simulink model "sine_dyn"  (R2022a)
settings: Solver=VariableStepAuto  StartTime=0.0  StopTime=12  MaxStep=0.05  RelTol=1e-3
libraries: simulink x2
settings Model: Creator=patri  LastModifiedBy=Mattia
settings SolverCC: ZeroCrossAlgorithm=Adaptive
settings DebuggingCC: IgnoredZcDiagnostic=none

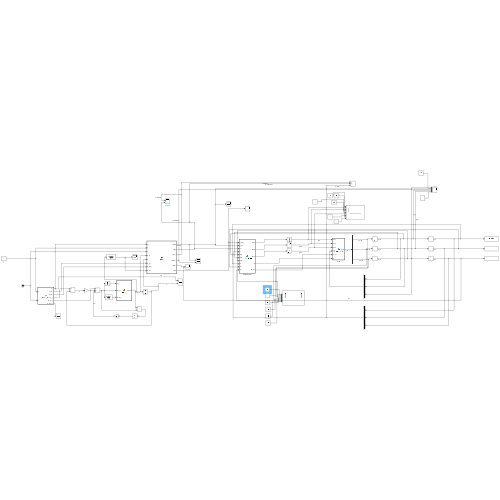
[thumbnail: Simulink's stored preview of the top-level diagram]
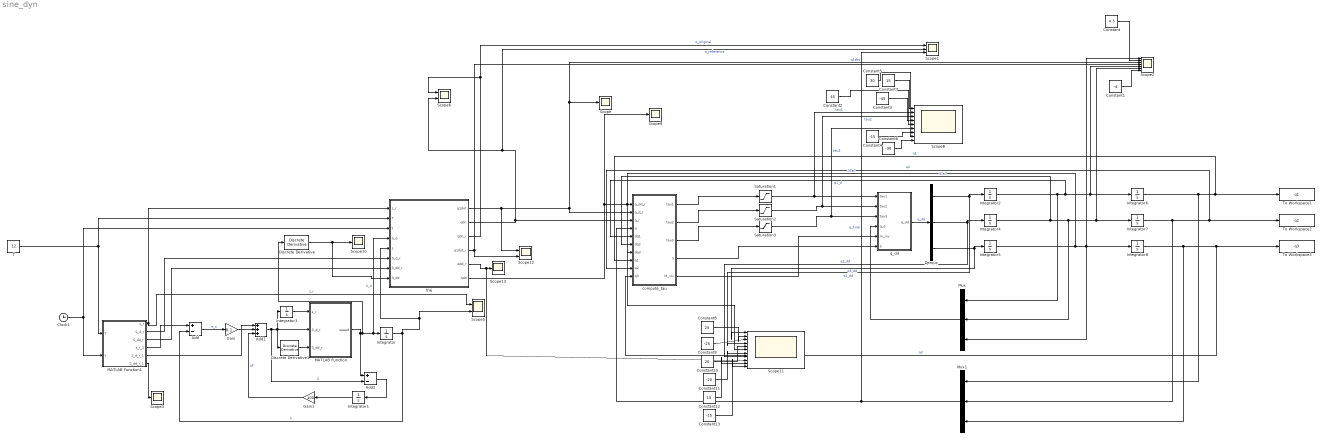
== system sine_dyn ==
  Add : Sum  Inputs=+-
  Add1 : Sum  Inputs=+++
  Add2 : Sum  Inputs=+-
  Clock1 : Clock
  Constant : Constant  Value=4.3
  Constant1 : Constant  Value=-4
  Constant10 : Constant  Value=20
  Constant11 : Constant  Value=-20
  Constant12 : Constant  Value=15
  Constant13 : Constant  Value=-15
  Constant2 : Constant  Value=45
  Constant3 : Constant  Value=-45
  Constant4 : Constant  Value=-15
  Constant5 : Constant  Value=30
  Constant6 : Constant  Value=-30
  Constant7 : Constant  Value=15
  Constant8 : Constant  Value=25
  Constant9 : Constant  Value=-25
  Demux : Demux  Outputs=3
  Discrete Derivative : simulink/Discrete/Discrete Derivative  gainval=1.0  ICPrevScaledInput=0.0  OutMin=[]  OutMax=[]  OutDataType=fixdt(1, 16)  OutScaling=2^-10  DoSatur=off
  Discrete Derivative1 : simulink/Discrete/Discrete Derivative  gainval=1.0  ICPrevScaledInput=0.0  OutMin=[]  OutMax=[]  OutDataType=fixdt(1, 16)  OutScaling=2^-10  DoSatur=off
  Gain : Gain  Gain=0.1
  Gain1 : Gain  Gain=100
  Integrator{,1..5} (6 alike) : Integrator
  Integrator6 : Integrator  InitialCondition=2.6180
  Integrator7 : Integrator  InitialCondition=-2.0944
  Integrator8 : Integrator  InitialCondition=-0.5236
  MATLAB Function : MATLAB Function  TreatAsAtomicUnit=on
  MATLAB Function1 : MATLAB Function  TreatAsAtomicUnit=on
  Mux : Mux  Inputs=3
  Mux1 : Mux  Inputs=3
  Saturation1 : Saturate  UpperLimit=45  LowerLimit=-45  LinearizeAsGain=off  ZeroCross=off
  Saturation2 : Saturate  UpperLimit=30  LowerLimit=-30  LinearizeAsGain=off  ZeroCross=off
  Saturation3 : Saturate  UpperLimit=15  LowerLimit=-15  LinearizeAsGain=off  ZeroCross=off
  Scope{,3,9..10,13} (5 alike) : Scope
  Scope1 : Scope  NumInputPorts=3
  Scope11 : Scope  NumInputPorts=11
  Scope12 : Scope  NumInputPorts=2
  Scope2 : Scope  NumInputPorts=7
  Scope5 : Scope  NumInputPorts=2
  Scope6 : Scope  NumInputPorts=2
  Scope8 : Scope  NumInputPorts=9
  T : Constant  Value=12
  To Workspace1 : ToWorkspace  VariableName=q1  SampleTime=-1
  To Workspace2 : ToWorkspace  VariableName=q2  SampleTime=-1
  To Workspace3 : ToWorkspace  VariableName=q3  SampleTime=-1
  compute_tau : MATLAB Function  TreatAsAtomicUnit=on
  q_dd : MATLAB Function  TreatAsAtomicUnit=on
  traj : MATLAB Function  TreatAsAtomicUnit=on
  wires:
  Demux/3 -> Integrator5/1, Scope11/1  "q3_dd"
  traj/2(q0n) -> compute_tau/3(q_r), Scope1/2, Scope6/2  "q_reference"
  Clock1/1 -> MATLAB Function1/2(t), traj/3(t)
  q_dd/1(q_dd) -> Demux/1  "q_dd"
  traj/3(q0n_r) -> Scope1/1, Scope6/1  "q_original"
  Add2/1 -> Integrator1/1
  Integrator4/1 -> compute_tau/6(dq2), Mux/2, Integrator7/1, Scope2/6  "q2_d"
  Integrator/1 -> traj/5(s), Scope5/2, Add/2  "s"
  compute_tau/4(S) -> q_dd/6(S)
  Integrator5/1 -> compute_tau/7(dq3), Scope2/1, Mux/3, Integrator8/1  "q3_d"
  Mux/1 -> q_dd/4(q_d)
  Demux/1 -> Integrator2/1, Scope11/4  "q1_dd"
  Mux1/1 -> Scope1/3, compute_tau/4(q)  "q_final"
  Integrator2/1 -> Mux/1, compute_tau/5(dq1), Scope2/5, Integrator6/1  "q1_d"
  Integrator6/1 -> Mux1/1, compute_tau/8(q1), To Workspace1/1  "q1"
  traj/6(qdd) -> Scope9/1, compute_tau/1(q_dd_r), Scope11/6
  MATLAB Function1/1(s_r) -> traj/1(s_r), Scope5/1  "s_r"
  Integrator8/1 -> Mux1/3, To Workspace3/1, compute_tau/10(q3)  "q3"
  traj/1(q1dot) -> Scope12/1, Scope2/3, Scope/1, compute_tau/2(q_d_r)  "q1dot"
  Gain/1 -> Add1/2
  compute_tau/5(M_inv) -> q_dd/5(m_inv)
  Add1/1 -> Add2/2, MATLAB Function/2(S_d_r), Discrete Derivative1/1, Integrator3/1  "U"
  T/1 -> MATLAB Function1/1(T), traj/2(T)
  MATLAB Function/1(speed) -> Add2/1, Discrete Derivative/1, traj/4(S_d), Integrator/1  "S_d"
  Add/1 -> Gain/1  "e_s"
  Gain1/1 -> Add1/3  "Uf"
  traj/4(q1dot_r) -> Scope2/4, Scope12/2
  Demux/2 -> Integrator4/1, Scope11/8  "q2_dd"
  Integrator1/1 -> Gain1/1
  Integrator7/1 -> Mux1/2, compute_tau/9(q2), To Workspace2/1  "q2"
  compute_tau/1(tau1) -> Saturation1/1
  Saturation1/1 -> Scope8/2, q_dd/1(tau1)  "tau1"
  compute_tau/2(tau2) -> Saturation2/1
  Saturation2/1 -> Scope8/3, q_dd/2(tau2)  "tau2"
  compute_tau/3(tau3) -> Saturation3/1
  Saturation3/1 -> Scope8/6, q_dd/3(tau3)  "tau3"
  Constant1/1 -> Scope2/7
  Constant/1 -> Scope2/2
  MATLAB Function1/2(S_d_r) -> traj/6(S_d_r)
  MATLAB Function1/3(S_dd_r) -> traj/7(S_dd_r)
  Constant4/1 -> Scope8/7
  Constant3/1 -> Scope8/4
  Constant7/1 -> Scope8/1
  Constant2/1 -> Scope8/5
  Discrete Derivative/1 -> Scope10/1, traj/8(S_dd)
  traj/5(qdd_r) -> Scope11/9, Scope13/1
  MATLAB Function1/4(s_r_1) -> Add/1
  MATLAB Function1/5(S_d_r_1) -> Add1/1
  MATLAB Function1/6(S_dd_r_1) -> Scope3/1
  Integrator3/1 -> MATLAB Function/1(s_r)
  Discrete Derivative1/1 -> MATLAB Function/3(S_dd_r)
  Constant5/1 -> Scope8/8
  Constant6/1 -> Scope8/9
  Constant8/1 -> Scope11/2
  Constant9/1 -> Scope11/3
  Constant10/1 -> Scope11/5
  Constant11/1 -> Scope11/7
  Constant12/1 -> Scope11/10
  Constant13/1 -> Scope11/11

== matlab function sine_dyn/q_dd ==
  data: tau1 input; tau2 input; tau3 input; q_dd output; q_d input; m_inv input; S input
function q_dd = compute_q_dd(tau1,tau2,tau3,q_d,m_inv,S)

tau = [tau1;
       tau2;
       tau3];
q_dd = m_inv*(tau - (S*q_d));

== matlab function sine_dyn/compute_tau ==
  data: q_dd_r input; tau1 output; tau2 output; tau3 output; q_d_r input; q_r input; q input; dq1 input; S output; M_inv output; dq2 input; dq3 input; q1 input; q2 input; q3 input
function [tau1,tau2,tau3,S,M_inv] = compute_tau(q_dd_r, q_d_r, q_r, q,dq1,dq2,dq3,q1,q2,q3)

% M(q)q_dd_r + S(q,q_d)q_d_r + Kp(q_r - q) + Kd (q_d_r - q_d)

% 
Kp = diag([0.1,0.1,0.1]);

Kd= diag([10,10,10]);

% 
%NEW GAIN TO STABILIZE ACCELERATION
% Kp = diag([30,30,30]);
% 
% Kd = diag([100,100,100]);

%%q

% q1=q_r(1);
% q2=q_r(2);
% q3=q_r(3);
% %%dq
% dq1=q_d_r(1);
% dq2=q_d_r(2);
% dq3=q_d_r(3);

q_d = [dq1;dq2;dq3];

%%position error
e = q_r - q;
%%velocity error
e_d = q_d_r - q_d;

L=1;

l1 = L;
l2 = L;
l3 = L;
dc1 = 1/2 * L;
dc2 = 1/2 * L;
dc3 = 1/2 * L;
m1 = 5;
m2 = 5;
m3 = 5;
I1 = 1/12 * m1 * L^2;
I2 = 1/12 * m2 * L^2;
I3 = 1/12 * m3 * L^2;

M=zeros(3,3);

M(1,1)=I1 + I2 + I3 + L^2*m2 + 2*L^2*m3 + 2*cos(q2)*(m3*L^2 + dc2*m2*L) + dc1^2*m1 + dc2^2*m2 + dc3^2*m3 + 2*L*dc3*m3*cos(q2 + q3) + 2*L*dc3*m3*cos(q3);
M(1,2)=I2 + I3 + L^2*m3 + cos(q2)*(m3*L^2 + dc2*m2*L) + dc2^2*m2 + dc3^2*m3 + L*dc3*m3*cos(q2 + q3) + 2*L*dc3*m3*cos(q3);
M(1,3)=I3 + dc3^2*m3 + L*dc3*m3*cos(q2 + q3) + L*dc3*m3*cos(q3);
M(2,2)=m3*L^2 + 2*m3*cos(q3)*L*dc3 + m2*dc2^2 + m3*dc3^2 + I2 + I3;
M(2,3)=m3*dc3^2 + L*m3*cos(q3)*dc3 + I3;
M(3,3)=m3*dc3^2 + I3;
M(2,1)=M(1,2);
M(3,1)=M(1,3);
M(3,2)=M(2,3);

M_inv = pinv(M);

S=zeros(3,3);

S(1,1) = -dq2*(dc3*l1*m3*sin(q2 + q3) + dc2*l1*m2*sin(q2) + l1*l2*m3*sin(q2)) - dq3*(dc3*l1*m3*sin(q2 + q3) + dc3*l2*m3*sin(q3));

S(1,2)= -dq1*(dc3*l1*m3*sin(q2 + q3) + dc2*l1*m2*sin(q2) + l1*l2*m3*sin(q2)) - dq2*(dc3*l1*m3*sin(q2 + q3) + dc2*l1*m2*sin(q2) + l1*l2*m3*sin(q2)) - dq3*(dc3*l1*m3*sin(q2 + q3) + dc3*l2*m3*sin(q3));

S(1,3)= -dq1*(dc3*l1*m3*sin(q2 + q3) + dc3*l2*m3*sin(q3)) - dq2*(dc3*l1*m3*sin(q2 + q3) + dc3*l2*m3*sin(q3)) - dq3*(dc3*l1*m3*sin(q2 + q3) + dc3*l2*m3*sin(q3)) ;

S(2,1)= dq1*(dc3*l1*m3*sin(q2 + q3) + dc2*l1*m2*sin(q2) + l1*l2*m3*sin(q2)) - dc3*dq3*l2*m3*sin(q3);

S(2,2)=-dc3*dq3*l2*m3*sin(q3);
 
S(2,3)= - dc3*dq1*l2*m3*sin(q3) - dc3*dq2*l2*m3*sin(q3) - dc3*dq3*l2*m3*sin(q3);

S(3,1)= dq1*(dc3*l1*m3*sin(q2 + q3) + dc3*l2*m3*sin(q3)) + dc3*dq2*l2*m3*sin(q3);

S(3,2)= dc3*dq1*l2*m3*sin(q3) + dc3*dq2*l2*m3*sin(q3);

S(3,3)= 0;


%torque = M*q_dd_r + S*q_d_r + Kp*e + Kd*e_d; %%viscous friction Fv*q_d_r
torque =M*q_dd_r + S*q_d_r + M*(Kp*e + Kd*e_d);

tau1 = torque(1);
tau2 = torque(2);
tau3 = torque(3);



%torque = M(q)*q_dd_r + S(q,q_d)*q_d_r + Kp*(q_r - q) + Kd*(q_d_r - q_d);

== matlab function sine_dyn/MATLAB Function1 ==
  data: T input; t input; s_r output; S_d_r output; S_dd_r output; s_r_1 output; S_d_r_1 output; S_dd_r_1 output
function [s_r, S_d_r, S_dd_r,s_r_1, S_d_r_1, S_dd_r_1] = timing_law(T, t)

tau_t=t/T;
%s_r = -2*tau_t^3 + 3*tau_t^2;
s_r = 10*tau_t^3 - 15*tau_t^4 + 6*tau_t^5;
S_d_r = (30*t^2)/T^3 - (60*t^3)/T^4 + (30*t^4)/T^5;
S_dd_r=(60*t)/T^3 - (180*t^2)/T^4 + (120*t^3)/T^5;
t_1 = t +0.0001;
tau_t_1 = t_1/T;
s_r_1 = 10*tau_t_1^3 - 15*tau_t_1^4 + 6*tau_t_1^5;
S_d_r_1 = (30*t_1^2)/T^3 - (60*t_1^3)/T^4 + (30*t_1^4)/T^5;
S_dd_r_1=(60*t_1)/T^3 - (180*t_1^2)/T^4 + (120*t_1^3)/T^5;

== matlab function sine_dyn/traj ==
  data: s_r input; T input; t input; S_d input; s input; q1dot output; q0n output; q0n_r output; q1dot_r output; S_d_r input; S_dd_r input; qdd_r output; qdd output; S_dd input
function [q1dot,q0n,q0n_r,q1dot_r, qdd_r, qdd] = trajectory(s_r, T, t, S_d, s, S_d_r, S_dd_r, S_dd)


%Links length
l1 = 1; l2 =1; l3 = 1;

%Trajectory

p_s = [s + 1;
    1 + sin(4*pi*s);
    s];

p_s_r =  [s_r + 1;
    1 + sin(4*pi*s_r);
    s_r];

p1_s=[1;
        4*pi*cos(4*pi*s);
        1];
p1_s_r=[1;
        4*pi*cos(4*pi*s_r);
        1];

%Velocity of the trajectory
pdot_s= p1_s* S_d ;
pdot_s_r = p1_s_r * S_d_r;
                                                                 

%End effector position
px = p_s(1); py = p_s(2); %position of the end effector w.r.t. the global frame

phi = p_s(3); %orientation of the end effector w.r.t. global frame

%%% REFERENCE

px_r=p_s_r(1); py_r = p_s_r(2);
phi_r = p_s_r(3);

%%Inverse kinematics of planar 3R
%fprintf("we first solve the joint variables q1, q2 in order to place\nthe position of the base of the third link in the necessary position\n");
 
p2 = [px; py] - [l3*cos(phi); l3*sin(phi)];
p2x = p2(1);
p2y = p2(2);

%%% REFERENCE

p2_r = [px_r; py_r] - [l3*cos(phi_r); l3*sin(phi_r)];
p2x_r = p2_r(1);
p2y_r = p2_r(2);

% second joint computations
c2=(p2x^2+p2y^2-l1^2-l2^2)/(2*l1*l2); s2pos=sqrt(1-c2^2);

%%% REFERENCE

c2_r=(p2x_r^2+p2y_r^2-l1^2-l2^2)/(2*l1*l2); s2pos_r=sqrt(1-c2_r^2);

%other solution: -sqrt(1-c2^2)
s2neg=-sqrt(1-c2^2);

q02p=atan2(s2pos,c2);
q02n=atan2(s2neg,c2);

%%% REFERENCE

s2neg_r=-sqrt(1-c2_r^2);

q02p_r=atan2(s2pos_r,c2_r);
q02n_r=atan2(s2neg_r,c2_r);
 
% first joint computations
detM=l1^2+l2^2+2*l1*l2*c2;

%%% REFERENCE

detM_r=l1^2+l2^2+2*l1*l2*c2_r;

% positive solution of q1
s1pos=(p2y*(l1+l2*c2)-p2x*l2*s2pos)/detM; c1pos=(p2x*(l1+l2*c2)+p2y*l2*s2pos)/detM;

%%% REFERENCE

s1pos_r=(p2y_r*(l1+l2*c2_r)-p2x_r*l2*s2pos_r)/detM_r; c1pos_r=(p2x_r*(l1+l2*c2_r)+p2y_r*l2*s2pos_r)/detM_r;

% negative solution of q1
s1neg=(p2y*(l1+l2*c2)-p2x*l2*s2neg)/detM;
c1neg=(p2x*(l1+l2*c2)+p2y*l2*s2neg)/detM;

q01p=atan2(s1pos,c1pos);
q01n=atan2(s1neg,c1neg); 

q03p = phi-(q01p+q02p);
q03n = phi-(q01n+q02n);

%%% REFERENCE

s1neg_r=(p2y_r*(l1+l2*c2_r)-p2x_r*l2*s2neg_r)/detM_r;
c1neg_r=(p2x_r*(l1+l2*c2_r)+p2y_r*l2*s2neg_r)/detM_r;

q01p_r=atan2(s1pos_r,c1pos_r);
q01n_r=atan2(s1neg_r,c1neg_r); 

q03p_r = phi_r-(q01p_r+q02p_r);
q03n_r = phi_r-(q01n_r+q02n_r);

% output positive
q0p=[q01p; q02p; q03p];

%%% REFERENCE

q0p_r=[q01p_r; q02p_r; q03p_r];
% output negative
q0n=[q01n; q02n; q03n];

%%% REFERENCE

q0n_r=[q01n_r; q02n_r; q03n_r];

%In a cubic polynomial the maximum of the speed of the timing law is
%obtained in t = T/2 
q1 = q0n(1);
q2 = q0n(2);
q3 = q0n(3);
P = [l1*cos(q1) + l2*cos(q1+q2) + l3*cos(q1+q2+q3);
    l1*sin(q1) + l2*sin(q1+q2) + l3*sin(q1+q2+q3)
    q1 + q2 + q3];

J = [- sin(q1 + q2 + q3) - sin(q1 + q2) - sin(q1), - sin(q1 + q2 + q3) - sin(q1 + q2), -sin(q1 + q2 + q3);
  cos(q1 + q2 + q3) + cos(q1 + q2) + cos(q1),   cos(q1 + q2 + q3) + cos(q1 + q2),  cos(q1 + q2 + q3);
                                          1,                                  1,                  1];

%%% REFERENCE

q1_r = q0n_r(1);
q2_r = q0n_r(2);
q3_r = q0n_r(3);
P_r = [l1*cos(q1_r) + l2*cos(q1_r+q2_r) + l3*cos(q1_r+q2_r+q3_r);
    l1*sin(q1_r) + l2*sin(q1_r+q2_r) + l3*sin(q1_r+q2_r+q3_r)
    q1 + q2 + q3];

J_r = [- sin(q1_r + q2_r + q3_r) - sin(q1_r + q2_r) - sin(q1_r), - sin(q1_r + q2_r + q3_r) - sin(q1_r + q2_r), -sin(q1_r + q2_r + q3_r);
  cos(q1_r + q2_r + q3_r) + cos(q1_r + q2_r) + cos(q1_r),   cos(q1_r + q2_r + q3_r) + cos(q1_r + q2_r),  cos(q1_r + q2_r + q3_r);
                                          1,                                  1,                  1];


qdot = pinv(J) * pdot_s;

%%% REFERENCE

qdot_r = pinv(J_r) * pdot_s_r;

q1dot = qdot;

q1dot_r = qdot_r;

dq1_r=qdot_r(1);
dq2_r=qdot_r(2);
dq3_r=qdot_r(3);
J_dot_r = [- cos(q1_r + q2_r + q3_r)*(dq1_r + dq2_r + dq3_r) - cos(q1_r + q2_r)*(dq1_r + dq2_r) - dq1_r*cos(q1_r), - cos(q1_r + q2_r + q3_r)*(dq1_r + dq2_r + dq3_r) - cos(q1_r + q2_r)*(dq1_r + dq2_r), -cos(q1_r + q2_r + q3_r)*(dq1_r + dq2_r + dq3_r);
           - sin(q1_r + q2_r + q3_r)*(dq1_r + dq2_r + dq3_r) - sin(q1_r + q2_r)*(dq1_r + dq2_r) - dq1_r*sin(q1_r), - sin(q1_r + q2_r + q3_r)*(dq1_r + dq2_r + dq3_r) - sin(q1_r + q2_r)*(dq1_r + dq2_r), -sin(q1_r + q2_r + q3_r)*(dq1_r + dq2_r + dq3_r) ;   
            0,0,0];
p2_s_r =[   0
-16*pi^2*sin(4*pi*s_r)
                     0];
p2_s =[   0
-16*pi^2*sin(4*pi*s)
                     0];
dq1=qdot(1);
dq2=qdot(2);
dq3=qdot(3);
J_dot = [- cos(q1 + q2 + q3)*(dq1 + dq2 + dq3) - cos(q1 + q2)*(dq1 + dq2) - dq1*cos(q1), - cos(q1 + q2 + q3)*(dq1 + dq2 + dq3) - cos(q1 + q2)*(dq1 + dq2), -cos(q1 + q2 + q3)*(dq1 + dq2 + dq3);
    - sin(q1 + q2 + q3)*(dq1 + dq2 + dq3) - sin(q1 + q2)*(dq1 + dq2) - dq1*sin(q1), - sin(q1 + q2 + q3)*(dq1 + dq2 + dq3) - sin(q1 + q2)*(dq1 + dq2), -sin(q1 + q2 + q3)*(dq1 + dq2 + dq3);
    0,0,0];

pdd_r = p1_s_r * S_dd_r + p2_s_r * S_d_r^2;

qdd_r = inv(J_r)*(pdd_r - J_dot_r*qdot_r);
pdd = p1_s * S_dd + p2_s * S_d^2;


qdd = inv(J)*(pdd - J_dot*qdot);

== matlab function sine_dyn/MATLAB Function ==
  data: s_r input; speed output; S_d_r input; S_dd_r input
function speed = trajectory(s_r, S_d_r,S_dd_r)

%Links length
l1 = 1; l2 =1; l3 = 1;

%Trajectory


%%% REFERENCE


p_s_r =  [s_r + 1;
    1 + sin(4*pi*s_r);
    s_r];

R1_s_r=[1;
        4*pi*cos(4*pi*s_r);
        1];

%Velocity of the trajectory


%%pdot = R'*s'(t)




%%% REFERENCE

%%%POLYNOMIAL OF DEGREE 5 ---  0.4808 saturation --- 3.9 seconds
% pdot_s_r=[ -(30*t^2*pi*sin((2*t^3*pi*(10*T^2 - 15*T*t + 6*t^2))/T^5)*(T - t)^2)/T^5;
%           (30*t^2*pi*cos((2*t^3*pi*(10*T^2 - 15*T*t + 6*t^2))/T^5)*(T - t)^2)/T^5;
%                                                                                 0];
pdot_s_r= R1_s_r* S_d_r ; %sdr is u
      

%%%%%%%%%%%%%%%%%%%
% pdot_s_r = [-pi*sin(2*pi*((10*t^3)/T^3 - (15*t^4)/T^4 + (6*t^5)/T^5))*((30*t^2)/T^3 - (60*t^3)/T^4 + (30*t^4)/T^5);
%  pi*cos(2*pi*((10*t^3)/T^3 - (15*t^4)/T^4 + (6*t^5)/T^5))*((30*t^2)/T^3 - (60*t^3)/T^4 + (30*t^4)/T^5);
%                                                                                                      0];

%End effector position

%%% REFERENCE

px_r=p_s_r(1); py_r = p_s_r(2);
phi_r = p_s_r(3);

%%Inverse kinematics of planar 3R, compute q

%%% REFERENCE

p2_r = [px_r; py_r] - [l3*cos(phi_r); l3*sin(phi_r)];
p2x_r = p2_r(1);
p2y_r = p2_r(2);

% second joint computations


%%% REFERENCE

c2_r=(p2x_r^2+p2y_r^2-l1^2-l2^2)/(2*l1*l2); s2pos_r=sqrt(1-c2_r^2);

%other solution: -sqrt(1-c2^2)

%%% REFERENCE

s2neg_r=-sqrt(1-c2_r^2);

q02p_r=atan2(s2pos_r,c2_r);
q02n_r=atan2(s2neg_r,c2_r);
 
% first joint computations


%%% REFERENCE

detM_r=l1^2+l2^2+2*l1*l2*c2_r;

% positive solution of q1


%%% REFERENCE

s1pos_r=(p2y_r*(l1+l2*c2_r)-p2x_r*l2*s2pos_r)/detM_r; c1pos_r=(p2x_r*(l1+l2*c2_r)+p2y_r*l2*s2pos_r)/detM_r;

% negative solution of q1


%%% REFERENCE

s1neg_r=(p2y_r*(l1+l2*c2_r)-p2x_r*l2*s2neg_r)/detM_r;
c1neg_r=(p2x_r*(l1+l2*c2_r)+p2y_r*l2*s2neg_r)/detM_r;

q01p_r=atan2(s1pos_r,c1pos_r);
q01n_r=atan2(s1neg_r,c1neg_r); 

q03p_r = phi_r-(q01p_r+q02p_r);
q03n_r = phi_r-(q01n_r+q02n_r);



%%% REFERENCE


% output negative


%%% REFERENCE

q0n_r=[q01n_r; q02n_r; q03n_r];
q1_r = q0n_r(1);
q2_r = q0n_r(2);
q3_r = q0n_r(3);

%NOW WE COMPUTE qdot, qdotdot

%%% REFERENCE


P_r = [l1*cos(q1_r) + l2*cos(q1_r+q2_r) + l3*cos(q1_r+q2_r+q3_r);
    l1*sin(q1_r) + l2*sin(q1_r+q2_r) + l3*sin(q1_r+q2_r+q3_r)
    q1_r + q2_r + q3_r];

J_r = [- sin(q1_r + q2_r + q3_r) - sin(q1_r + q2_r) - sin(q1_r), - sin(q1_r + q2_r + q3_r) - sin(q1_r + q2_r), -sin(q1_r + q2_r + q3_r);
  cos(q1_r + q2_r + q3_r) + cos(q1_r + q2_r) + cos(q1_r),   cos(q1_r + q2_r + q3_r) + cos(q1_r + q2_r),  cos(q1_r + q2_r + q3_r);
                                          1,                                  1,                  1];


qdot_r = pinv(J_r) * pdot_s_r;

dq1_r=qdot_r(1);
dq2_r=qdot_r(2);
dq3_r=qdot_r(3);
J_dot_r = [- cos(q1_r + q2_r + q3_r)*(dq1_r + dq2_r + dq3_r) - cos(q1_r + q2_r)*(dq1_r + dq2_r) - dq1_r*cos(q1_r), - cos(q1_r + q2_r + q3_r)*(dq1_r + dq2_r + dq3_r) - cos(q1_r + q2_r)*(dq1_r + dq2_r), -cos(q1_r + q2_r + q3_r)*(dq1_r + dq2_r + dq3_r);
           - sin(q1_r + q2_r + q3_r)*(dq1_r + dq2_r + dq3_r) - sin(q1_r + q2_r)*(dq1_r + dq2_r) - dq1_r*sin(q1_r), - sin(q1_r + q2_r + q3_r)*(dq1_r + dq2_r + dq3_r) - sin(q1_r + q2_r)*(dq1_r + dq2_r), -sin(q1_r + q2_r + q3_r)*(dq1_r + dq2_r + dq3_r) ;   
            0,0,0];

%directly calculated
% pdd_r = [pi*sin(2*pi*((10*t^3)/T^3 - (15*t^4)/T^4 + (6*t^5)/T^5))*((60*t)/T^3 - (180*t^2)/T^4 + (120*t^3)/T^5) - 2*pi^2*cos(2*pi*((10*t^3)/T^3 - (15*t^4)/T^4 + (6*t^5)/T^5))*((30*t^2)/T^3 - (60*t^3)/T^4 + (30*t^4)/T^5)^2;
%        pi*cos(2*pi*((10*t^3)/T^3 - (15*t^4)/T^4 + (6*t^5)/T^5))*((60*t)/T^3 - (180*t^2)/T^4 + (120*t^3)/T^5) - 2*pi^2*sin(2*pi*((10*t^3)/T^3 - (15*t^4)/T^4 + (6*t^5)/T^5))*((30*t^2)/T^3 - (60*t^3)/T^4 + (30*t^4)/T^5)^2;
%         0];
 %%(60*t)/T^3 - (180*t^2)/T^4 + (120*t^3)/T^5

q1d_r=dq1_r;
q2d_r=dq2_r;
q3d_r=dq3_r;

pdotdot_s_r =[   0
        -16*pi^2*sin(4*pi*s_r)
                     0];

pdd_r = R1_s_r * S_dd_r + pdotdot_s_r * S_d_r^2;

qdd_r = inv(J_r)*(pdd_r - J_dot_r*qdot_r);

q1dd_r=qdd_r(1);
q2dd_r=qdd_r(2);
q3dd_r=qdd_r(3);
%%%%%%%%%%%%%%%%%%%%%%%%%%%%%%%%%%%%%%%%%%%%%%%%%%%%%%%%%%%%
%%bounds
q1_max=3.5;   q1_min=-3.5;
q2_max=3;     q2_min=-3;
q3_max= 2.57; q2_min =-2.57;
q1d_max= 4;   q1d_min=-4;
q2d_max=4;    q2d_min = -4;
q3d_max=4.3;  q3d_min=-4.3;
q1dd_max=20;  q1dd_min=-20;
q2dd_max=15;  q2dd_min=-15;
q3dd_max=20;  q3dd_min=-20;


constraint_pos = max([abs(q1_r/q1_max); abs(q2_r/q2_max);abs(q3_r/q3_max)]);

constraint_vel = max([abs(q1d_r/q1d_max);abs(q2d_r/q2d_max);abs(q3d_r/q3d_max)]);

constraint_acc = max([abs(q1dd_r/q1dd_max); abs(q2dd_r/q2dd_max);abs(q3dd_r/q3dd_max)]);

most_constrained = max([1;constraint_vel;(constraint_acc)]);

speed = S_d_r / most_constrained;
